simulink model "magLev_sim"  (R2016b)
settings: Solver=ode4  StartTime=0.0  StopTime=T  FixedStep=ts  RelTol=1e-3
values from neighbouring files (symbols this model uses):
  A = full(A_fun(xeq,ueq))    [main.m]
  B = full(B_fun(xeq,ueq))    [main.m]
  GainScheduling = Simulink.Parameter(GainScheduling)    [main.m]
  sys = ss(A,B,C,D,      'name'     ,['Mag Lev trimmed p = ',num2str(position),' [m]'],      'StateName',{'p','v','i'},      'StateUnit',{'[m]','[m/s]','[A]'},      'InputName',{'V'},      'InputUnit',{'Volt'},      'OutputName',{'p'},      'OutputUnit',{'[m]'})    [main.m]
  SystemCompensated = ss(Phi,G,H,L,      'name'     ,'Mag Lev + LQI',      'StateName',{'p','v','i','ep'},      'StateUnit',{'[m]','[m/s]','[A]','[m]'},      'InputName',{'p'},      'InputUnit',{'[p]'},      'OutputName',{'p','u'},      'OutputUnit',{'[m]','[V]'})    [main.m]
  trimPoint = struct    [main.m]
  ts = 0.01    [main.m]
undefined symbols (not defined in the file or in its folder): Kfb, Kff
settings Model: Creator=Gianni  LastModifiedBy=Gianni

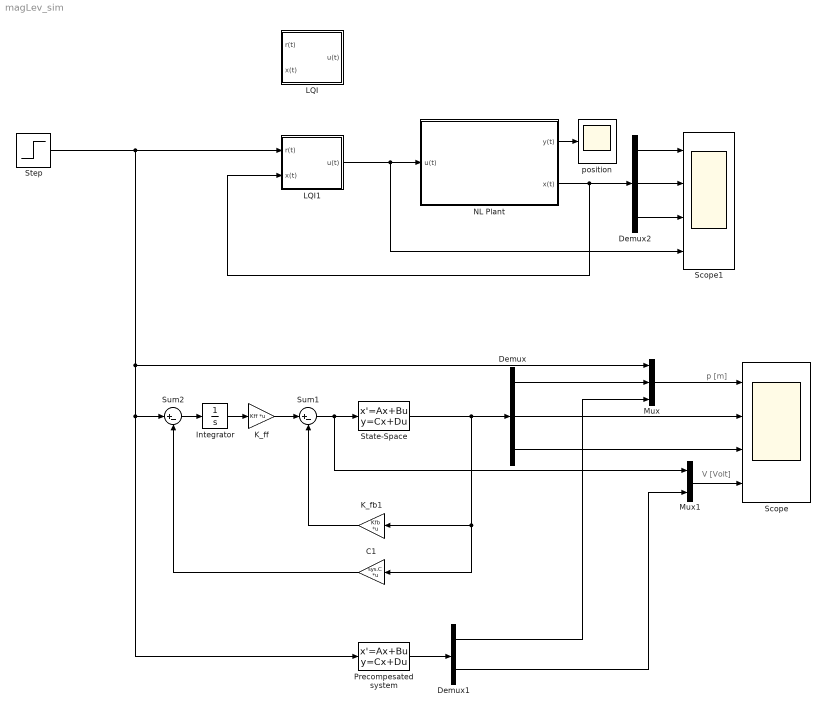
== system magLev_sim ==
  note: p [m]
  note: V [Volt]
  C1 : Gain  Gain=sys.C  Multiplication=Matrix(K*u)
  Demux : Demux  Outputs=3
  Demux1 : Demux  Outputs=2
  Demux2 : Demux  Outputs=3
  Integrator : Integrator
  K_fb1 : Gain  Gain=Kfb  Multiplication=Matrix(K*u)
  K_ff : Gain  Gain=Kff  Multiplication=Matrix(K*u)
  LQI : Subsystem
  LQI1 : Subsystem
  Mux : Mux  Inputs=3
  Mux1 : Mux  Inputs=2
  NL Plant : Subsystem
  Precompesated system : StateSpace  A=SystemCompensated.A  B=SystemCompensated.B  C=SystemCompensated.C  D=SystemCompensated.D  X0=0
  Scope : Scope  NumInputPorts=4
  Scope1 : Scope  NumInputPorts=4
  State-Space : StateSpace  A=sys.A  B=sys.B  C=eye(length(A))  D=zeros(size(B))  X0=0
  Step : Step  SampleTime=0
  Sum1 : Sum  Inputs=|+-
  Sum2 : Sum  Inputs=|+-
  position : Scope
  wires:
  Sum1/1 -> Mux1/1, State-Space/1
  K_fb1/1 -> Sum1/2
  C1/1 -> Sum2/2
  Sum2/1 -> Integrator/1
  Integrator/1 -> K_ff/1
  K_ff/1 -> Sum1/1
  State-Space/1 -> Demux/1, C1/1, K_fb1/1
  Demux/1 -> Mux/2
  Mux/1 -> Scope/1
  Demux/2 -> Scope/2
  Demux/3 -> Scope/3
  Mux1/1 -> Scope/4
  Precompesated system/1 -> Demux1/1
  Demux1/1 -> Mux/3
  Demux1/2 -> Mux1/2
  Demux2/1 -> Scope1/1
  Demux2/2 -> Scope1/2
  Demux2/3 -> Scope1/3
  NL Plant/2(x(t)) -> LQI1/2(x(t)), Demux2/1
  NL Plant/1(y(t)) -> position/1
  Step/1 -> LQI1/1(r(t)), Precompesated system/1, Sum2/1, Mux/1
  LQI1/1(u(t)) -> Scope1/4, NL Plant/1(u(t))

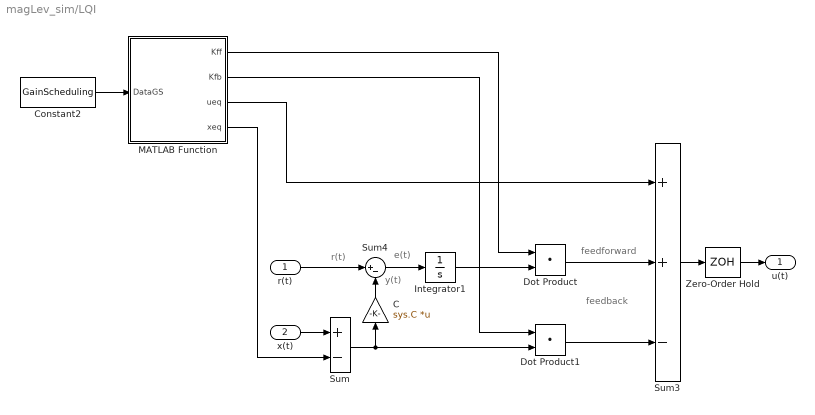
== system magLev_sim/LQI ==
  note: feedforward
  note: feedback
  note: e(t)
  note: y(t)
  note: r(t)
  r(t) : Inport
  x(t) : Inport  Port=2
  C : Gain  Gain=sys.C  Multiplication=Matrix(K*u)
  Constant2 : Constant  Value=GainScheduling  OutDataTypeStr=Bus: GainSchedulingStruct
  Dot Product : DotProduct  InputSameDT=on  OutDataTypeStr=Inherit: Inherit via internal rule
  Dot Product1 : DotProduct  InputSameDT=on  OutDataTypeStr=Inherit: Inherit via internal rule
  Integrator1 : Integrator
  MATLAB Function : MATLAB Function  TreatAsAtomicUnit=on
  Sum : Sum  Inputs=+-
  Sum3 : Sum  Inputs=++-
  Sum4 : Sum  Inputs=|+-
  Zero-Order Hold : ZeroOrderHold  SampleTime=ts
  u(t) : Outport
  wires:
  C/1 -> Sum4/2
  Sum4/1 -> Integrator1/1
  Integrator1/1 -> Dot Product/2
  Sum3/1 -> Zero-Order Hold/1
  r(t)/1 -> Sum4/1
  x(t)/1 -> Sum/1
  Dot Product1/1 -> Sum3/3
  Constant2/1 -> MATLAB Function/1(DataGS)
  Dot Product/1 -> Sum3/2
  MATLAB Function/2(Kfb) -> Dot Product1/1
  MATLAB Function/3(ueq) -> Sum3/1
  MATLAB Function/1(Kff) -> Dot Product/1
  Sum/1 -> C/1, Dot Product1/2
  MATLAB Function/4(xeq) -> Sum/2
  Zero-Order Hold/1 -> u(t)/1

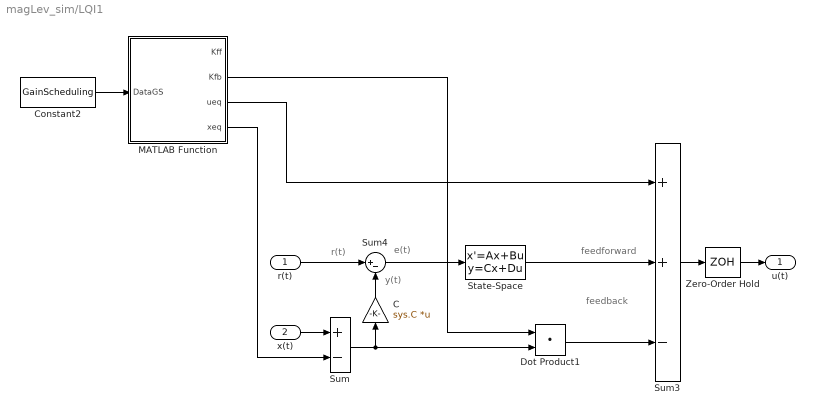
== system magLev_sim/LQI1 ==
  note: feedforward
  note: feedback
  note: e(t)
  note: y(t)
  note: r(t)
  r(t) : Inport
  x(t) : Inport  Port=2
  C : Gain  Gain=sys.C  Multiplication=Matrix(K*u)
  Constant2 : Constant  Value=GainScheduling  OutDataTypeStr=Bus: GainSchedulingStruct
  Dot Product1 : DotProduct  InputSameDT=on  OutDataTypeStr=Inherit: Inherit via internal rule
  MATLAB Function : MATLAB Function  TreatAsAtomicUnit=on
  State-Space : StateSpace  A=0  B=8  C=-6.355  D=0  X0=0
  Sum : Sum  Inputs=+-
  Sum3 : Sum  Inputs=++-
  Sum4 : Sum  Inputs=|+-
  Zero-Order Hold : ZeroOrderHold  SampleTime=ts
  u(t) : Outport
  wires:
  C/1 -> Sum4/2
  Sum4/1 -> State-Space/1
  Sum3/1 -> Zero-Order Hold/1
  r(t)/1 -> Sum4/1
  x(t)/1 -> Sum/1
  Dot Product1/1 -> Sum3/3
  Constant2/1 -> MATLAB Function/1(DataGS)
  State-Space/1 -> Sum3/2
  MATLAB Function/2(Kfb) -> Dot Product1/1
  MATLAB Function/3(ueq) -> Sum3/1
  Sum/1 -> C/1, Dot Product1/2
  MATLAB Function/4(xeq) -> Sum/2
  Zero-Order Hold/1 -> u(t)/1

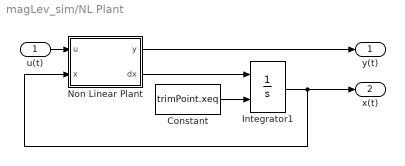
== system magLev_sim/NL Plant ==
  u(t) : Inport
  Constant : Constant  Value=trimPoint.xeq
  Integrator1 : Integrator  InitialConditionSource=external  InitialCondition=trimPoint.xeq
  Non Linear Plant : MATLAB Function  TreatAsAtomicUnit=on
  y(t) : Outport
  x(t) : Outport  Port=2
  wires:
  u(t)/1 -> Non Linear Plant/1(u)
  Non Linear Plant/1(y) -> y(t)/1
  Integrator1/1 -> x(t)/1, Non Linear Plant/2(x)
  Constant/1 -> Integrator1/2
  Non Linear Plant/2(dx) -> Integrator1/1

== matlab function magLev_sim/LQI/MATLAB Function ==
  data: DataGS input; Kff output; Kfb output; ueq output; xeq output
function [Kff,Kfb,ueq,xeq] = fcn(DataGS)
    Kff = DataGS.Kff;
    Kfb = DataGS.Kfb;
    xeq = DataGS.xeq;
    ueq = DataGS.ueq;
end

== matlab function magLev_sim/NL Plant/Non Linear Plant ==
  data: u input; y output; x input; dx output
function [y,dx] = MagLev(u,x)

    g0 = 9.81;  R = 50;    L = 0.5;
    m  = 0.02; Km = 19.62; b = 0.1;
     
    x1 = x(1); % position [m]
    x2 = x(2); % velocity [m/s]
    x3 = x(3); % current  [A]

    %u % voltage  [V]

    dx = [x2;
          g0-(b/m)*x2-(Km/m)*((x3/x1)^2);
         (1/(L+Km/x1))*(-R*x3+Km*(x2/(x1^2))+u)];  
      y = x1;
end

== matlab function magLev_sim/LQI1/MATLAB Function ==
  data: DataGS input; Kff output; Kfb output; ueq output; xeq output
function [Kff,Kfb,ueq,xeq] = fcn(DataGS)
    Kff = DataGS.Kff;
    Kfb = DataGS.Kfb;
    xeq = DataGS.xeq;
    ueq = DataGS.ueq;
end
